simulink model "LQR_forRTMaps10ms"  (R2024a)
settings: Solver=FixedStepAuto  StartTime=0.0  StopTime=10.0  FixedStep=0.01  RelTol=1e-3
settings Model: Creator=darkh  LastModifiedBy=darkh
settings OptimizationCC: ZeroExternalMemoryAtStartup=off  ZeroInternalMemoryAtStartup=off
settings RTWCC: Description=Generate an RTMaps component embedding the model  SystemTargetFile=rtmaps.tlc  TemplateMakefile=rtmaps_default_tmf  PostCodeGenCommand=rtmaps_post_code_generation(buildInfo)  RetainRTWFile=on  TargetLang=C++
settings STFCustomTargetCC: TargetLangStandard=C++11 (ISO)  ModelReferenceCompliant=off  ConcurrentExecutionCompliant=on  CombineOutputUpdateFcns=on  CodeInterfacePackaging=C++ class  CPPClassGenCompliant=on  GRTInterface=off  UseToolchainInfoCompliant=off  SystemTargetFile=rtmaps.tlc
settings GRTTargetCC: TargetLangStandard=C++11 (ISO)  ModelReferenceCompliant=off  ParMdlRefBuildCompliant=off  CompOptLevelCompliant=off  MatFileLogging=off  CodeInterfacePackaging=C++ class  UseToolchainInfoCompliant=off

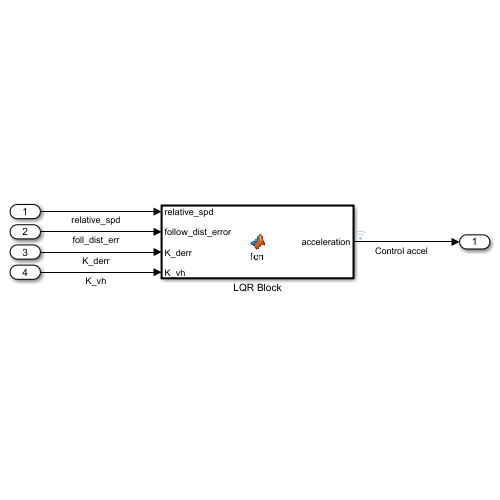
[thumbnail: Simulink's stored preview of the top-level diagram]
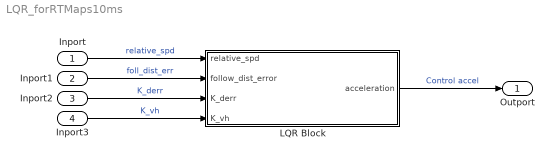
== system LQR_forRTMaps10ms ==
  Inport : Inport
  Inport1 : Inport  Port=2
  Inport2 : Inport  Port=3
  Inport3 : Inport  Port=4
  LQR Block : MATLAB Function  TreatAsAtomicUnit=on
  Outport : Outport
  wires:
  Inport/1 -> LQR Block/1(relative_spd)  "relative_spd"
  Inport1/1 -> LQR Block/2(follow_dist_error)  "foll_dist_err"
  Inport2/1 -> LQR Block/3(K_derr)  "K_derr"
  Inport3/1 -> LQR Block/4(K_vh)  "K_vh"
  LQR Block/1(acceleration) -> Outport/1  "Control accel"

== matlab function LQR_forRTMaps10ms/LQR Block ==
  data: relative_spd input; acceleration output; follow_dist_error input; K_derr input; K_vh input
function acceleration = fcn(relative_spd, follow_dist_error, K_derr, K_vh)
u = -K_derr*follow_dist_error-K_vh*relative_spd;
acceleration = u;
